simulink model "SMC_ISTSMC_ATSMC_IASMC_Leukemia_nonmono"  (R2024b)
settings: Solver=VariableStepAuto  StartTime=0.0  StopTime=20  RelTol=1e-3  EnableMultiTasking=on
undefined symbols (not defined in the file or in its folder): DiscIntNeverNeededParam
settings Model: Creator=engry  LastModifiedBy=munir
settings SolverCC: DateTimeAtSimulationTimeZero=[]  AlgebraicLoopSolver=TrustRegion
settings DataIOCC: ReturnWorkspaceOutputs=off
settings OptimizationCC: LifeSpan=inf
settings DebuggingCC: UnconnectedInputMsg=warning  UnconnectedOutputMsg=warning  UnconnectedLineMsg=warning  SFUnexpectedBacktrackingDiag=warning  SFNoUnconditionalDefaultTransitionDiag=warning  ArithmeticOperatorsInVariantConditions=warning
settings ModelReferenceCC: EnableRefExpFcnMdlSchedulingChecks=on
settings SFSimCC: SimUseLocalCustomCode=off  CustomCodeUndefinedFunction=UseInterfaceOnly
settings RTWCC: RTWUseLocalCustomCode=off  GPUComputeCapability=3.5
settings CodeAppCC: StateflowObjectComments=on
settings GRTTargetCC: TargetLangStandard=C89/C90 (ANSI)
settings ConfigComp: CovMetricSettings=dw  CovSaveCumulativeToWorkspaceVar=on  CovSaveSingleToWorkspaceVar=on  CovExternalEMLEnable=off

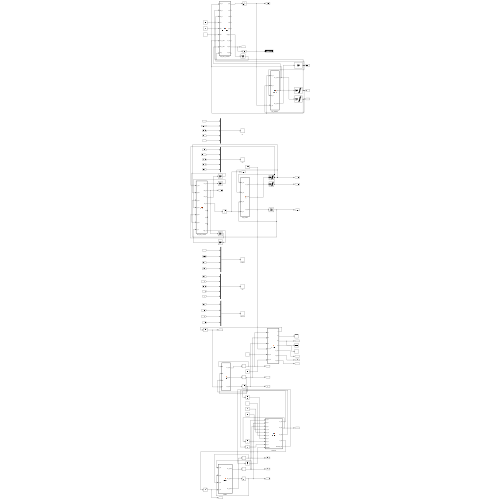
[thumbnail: Simulink's stored preview of the top-level diagram]
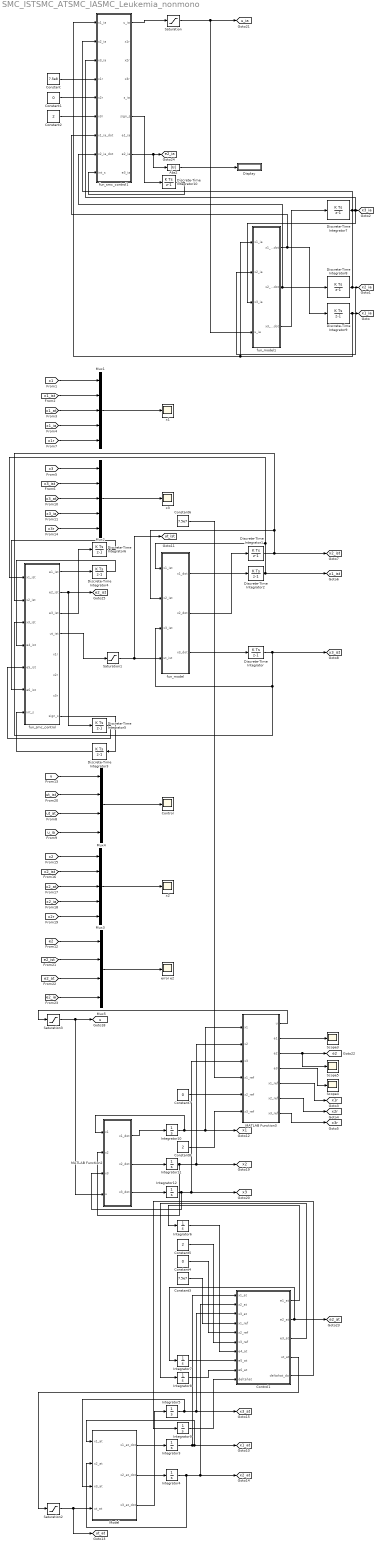
== system SMC_ISTSMC_ATSMC_IASMC_Leukemia_nonmono ==
  Abs2 : Abs  SaturateOnIntegerOverflow=off
  Constant : Constant  Value=7.5e8
  Constant1 : Constant  Value=0
  Constant2 : Constant  Value=2
  Constant3 : Constant  Value=7.5e7
  Constant4 : Constant  Value=0
  Constant5 : Constant  Value=2
  Constant6 : Constant  Value=7.5e7
  Constant7 : Constant  Value=0
  Constant8 : Constant  Value=2
  Control : Scope
  Control1 : MATLAB Function  TreatAsAtomicUnit=on  SystemSampleTime=0.01
  Discrete-Time Integrator : DiscreteIntegrator  SampleTime=-1  LowerSaturationLimit=0  ICPrevOutput=DiscIntNeverNeededParam  ICPrevScaledInput=DiscIntNeverNeededParam
  Discrete-Time Integrator1 : DiscreteIntegrator  InitialCondition=1e8  SampleTime=-1  LimitOutput=on  LowerSaturationLimit=0  ICPrevOutput=DiscIntNeverNeededParam  ICPrevScaledInput=DiscIntNeverNeededParam
  Discrete-Time Integrator10 : DiscreteIntegrator  SampleTime=-1  LowerSaturationLimit=0  ICPrevOutput=DiscIntNeverNeededParam  ICPrevScaledInput=DiscIntNeverNeededParam
  Discrete-Time Integrator2 : DiscreteIntegrator  InitialCondition=1.8e8  SampleTime=-1  LimitOutput=on  LowerSaturationLimit=7.5e7  ICPrevOutput=DiscIntNeverNeededParam  ICPrevScaledInput=DiscIntNeverNeededParam
  Discrete-Time Integrator{3..6} (4 alike) : DiscreteIntegrator  SampleTime=-1  ICPrevOutput=DiscIntNeverNeededParam  ICPrevScaledInput=DiscIntNeverNeededParam
  Discrete-Time Integrator7 : DiscreteIntegrator  SampleTime=-1  UpperSaturationLimit=2  LowerSaturationLimit=0  ICPrevOutput=DiscIntNeverNeededParam  ICPrevScaledInput=DiscIntNeverNeededParam
  Discrete-Time Integrator8 : DiscreteIntegrator  InitialCondition=1e8  SampleTime=-1  LimitOutput=on  LowerSaturationLimit=0  ICPrevOutput=DiscIntNeverNeededParam  ICPrevScaledInput=DiscIntNeverNeededParam
  Discrete-Time Integrator9 : DiscreteIntegrator  InitialCondition=1.8e8  SampleTime=-1  LimitOutput=on  LowerSaturationLimit=7.5e7  ICPrevOutput=DiscIntNeverNeededParam  ICPrevScaledInput=DiscIntNeverNeededParam
  Display : Display
  Integrator10 : Integrator  InitialCondition=1e8  LimitOutput=on  LowerSaturationLimit=7.5e7
  Integrator11 : Integrator  InitialCondition=1.8e8  LimitOutput=on  LowerSaturationLimit=0
  Integrator12 : Integrator  LimitOutput=on  UpperSaturationLimit=2  LowerSaturationLimit=0
  Integrator3 : Integrator  InitialCondition=1.8e8  LimitOutput=on  LowerSaturationLimit=7.5e7  ZeroCross=off
  Integrator4 : Integrator  InitialCondition=1e8  LimitOutput=on  LowerSaturationLimit=0
  Integrator5 : Integrator  ZeroCross=off
  Integrator{6..9} (4 alike) : Integrator
  MATLAB Function2 : MATLAB Function  TreatAsAtomicUnit=on
  MATLAB Function3 : MATLAB Function  TreatAsAtomicUnit=on
  Model : MATLAB Function  TreatAsAtomicUnit=on
  Mux1 : Mux  Inputs=5
  Mux2 : Mux  Inputs=5
  Mux3 : Mux  Inputs=5
  Mux4 : Mux
  Mux5 : Mux
  Saturation : Saturate  UpperLimit=1  LowerLimit=0
  Saturation1 : Saturate  UpperLimit=1  LowerLimit=0
  Saturation2 : Saturate  UpperLimit=1  LowerLimit=0  ZeroCross=off  RndMeth=Ceiling
  Saturation3 : Saturate  UpperLimit=1  LowerLimit=0  ZeroCross=off  RndMeth=Ceiling
  Scope3 : Scope
  Scope4 : Scope
  Scope5 : Scope
  error e2 : Scope
  fun_model : MATLAB Function  TreatAsAtomicUnit=on
  fun_model1 : MATLAB Function  TreatAsAtomicUnit=on
  fun_smc_control : MATLAB Function  TreatAsAtomicUnit=on
  fun_smc_control1 : MATLAB Function  TreatAsAtomicUnit=on
  x1 : Scope
  x2 : Scope
  x3 : Scope
  tag scope: e2=global, e2_at=global, e2_ia=global, e2_ist=global, u=global, u_ia=global, ut_at=global, ut_ist=global, x1=global, x1_at=global, x1_ia=global, x1_ist=global, x1r=global, x2=global, x2_at=global, x2_ia=global, x2_ist=global, x2r=global, x3=global, x3_at=global, x3_ia=global, x3_ist=global, x3r=global
  wires:
  Constant/1 -> fun_smc_control1/4("x1r ")
  Saturation2/1 -> [ut_at], Model/4(ut_at)
  fun_model/1(x1_dot) -> Discrete-Time Integrator2/1
  [x3_ia] -> Mux2/4
  Integrator7/1 -> Control1/8(e5_at)
  [x1] -> Mux1/1
  fun_model/3(x3_dot) -> Discrete-Time Integrator/1
  Constant1/1 -> fun_smc_control1/5("x2r ")
  Constant6/1 -> MATLAB Function3/4("x1_ref ")
  Constant2/1 -> fun_smc_control1/6("x3r ")
  Mux2/1 -> x3/1
  fun_smc_control/8(sign_s) -> Discrete-Time Integrator3/1
  [x3r] -> Mux2/5
  [x1_ist] -> Mux1/2
  [e2_at] -> Mux5/3
  [x1_at] -> Mux1/3
  [e2_ia] -> Mux5/4
  [x1_ia] -> Mux1/4
  Control1/5(deltahat_dot) -> Integrator9/1
  [u_ia] -> Mux4/4
  [x1r] -> Mux1/5
  [ut_ist] -> Mux4/2
  [x3] -> Mux2/1
  Integrator10/1 -> MATLAB Function3/1(x1), [x1], MATLAB Function2/1(x1)
  [x3_ist] -> Mux2/2
  [e2] -> Mux5/1
  [x3_at] -> Mux2/3
  fun_smc_control1/6(sign_s) -> Discrete-Time Integrator10/1
  fun_smc_control/1(e1_ist) -> Discrete-Time Integrator4/1
  [e2_ist] -> Mux5/2
  fun_smc_control/2(e2_ist) -> [e2_ist], Discrete-Time Integrator5/1
  fun_smc_control/3(e3_ist) -> Discrete-Time Integrator6/1
  fun_smc_control/4(ut_ist) -> Saturation1/1
  [u] -> Mux4/1
  Mux4/1 -> Control/1
  Discrete-Time Integrator4/1 -> fun_smc_control/4(e4_ist)
  [x2] -> Mux3/1
  [x2r] -> Mux3/5
  MATLAB Function3/2(e1) -> Scope3/1
  [ut_at] -> Mux4/3
  Saturation1/1 -> [ut_ist], fun_model/4(ut_ist)
  Discrete-Time Integrator6/1 -> fun_smc_control/6(e6_ist)
  [x2_ia] -> Mux3/4
  [x2_ist] -> Mux3/2
  [x2_at] -> Mux3/3
  Discrete-Time Integrator5/1 -> fun_smc_control/5(e5_ist)
  Saturation3/1 -> MATLAB Function2/4(u), [u]
  Mux5/1 -> error e2/1
  Discrete-Time Integrator3/1 -> fun_smc_control/7(int_s)
  Saturation/1 -> fun_model1/4(u_ia), [u_ia]
  fun_smc_control1/1(u_ia) -> Saturation/1
  Mux3/1 -> x2/1
  fun_smc_control1/8(e2_ia) -> [e2_ia], Abs2/1
  Discrete-Time Integrator10/1 -> fun_smc_control1/9(int_s)
  Mux1/1 -> x1/1
  MATLAB Function2/1(x1_dot) -> Integrator10/1
  MATLAB Function2/2(x2_dot) -> Integrator11/1
  Integrator9/1 -> Control1/10(deltahat)
  MATLAB Function2/3(x3_dot) -> Integrator12/1
  Model/1(x1_at_dot) -> Integrator3/1
  Model/2(x2_at_dot) -> Integrator4/1
  Constant7/1 -> MATLAB Function3/5("x2_ref ")
  Model/3(x3_at_dot) -> Integrator5/1
  Abs2/1 -> Display/1
  fun_model/2(x2_dot) -> Discrete-Time Integrator1/1
  Constant8/1 -> MATLAB Function3/6("x3_ref ")
  Integrator11/1 -> MATLAB Function3/2(x2), [x2], MATLAB Function2/2(x2)
  Integrator12/1 -> MATLAB Function3/3(x3), [x3], MATLAB Function2/3(x3)
  Integrator6/1 -> Control1/7(e4_at)
  Constant5/1 -> Control1/6(x3_ref)
  Constant4/1 -> Control1/5(x2_ref)
  Constant3/1 -> Control1/4(x1_ref)
  Integrator8/1 -> Control1/9(e6_at)
  MATLAB Function3/4(e3) -> Scope4/1
  Integrator5/1 -> [x3_at], Control1/3(x3_at), Model/3(x3_at)
  Integrator3/1 -> Model/1(x1_at), [x1_at], Control1/1(x1_at)
  Integrator4/1 -> [x2_at], Control1/2(x2_at), Model/2(x2_at)
  fun_model1/1(x1_ia_dot) -> fun_smc_control1/7(x1_ia_dot), Discrete-Time Integrator9/1
  fun_model1/2(x2_ia_dot) -> fun_smc_control1/8(x2_ia_dot), Discrete-Time Integrator8/1
  fun_model1/3(x3_ia_dot) -> Discrete-Time Integrator7/1
  Discrete-Time Integrator1/1 -> fun_smc_control/2(x2_ist), fun_model/2(x2_ist), [x2_ist]
  Discrete-Time Integrator2/1 -> fun_model/1(x1_ist), fun_smc_control/1(x1_ist), [x1_ist]
  Discrete-Time Integrator/1 -> fun_smc_control/3(x3_ist), fun_model/3(x3_ist), [x3_ist]
  MATLAB Function3/1(u) -> Saturation3/1
  MATLAB Function3/3(e2) -> [e2], Scope5/1
  MATLAB Function3/5(x1_ref) -> [x1r]
  MATLAB Function3/6(x2_ref) -> [x2r]
  MATLAB Function3/7(x3_ref) -> [x3r]
  Control1/1(e1_at) -> Integrator6/1
  Control1/2(e2_at) -> Integrator7/1, [e2_at]
  Control1/3(e3_at) -> Integrator8/1
  Control1/4(ut_at) -> Saturation2/1
  Discrete-Time Integrator7/1 -> fun_smc_control1/3(x3_ia), fun_model1/3(x3_ia), [x3_ia]
  Discrete-Time Integrator8/1 -> fun_smc_control1/2(x2_ia), [x2_ia], fun_model1/2(x2_ia)
  Discrete-Time Integrator9/1 -> fun_model1/1(x1_ia), fun_smc_control1/1(x1_ia), [x1_ia]

== matlab function SMC_ISTSMC_ATSMC_IASMC_Leukemia_nonmono/Model ==
  data: x1_at input; x1_at_dot output; x2_at input; x3_at input; x2_at_dot output; x3_at_dot output; ut_at input
function[x1_at_dot, x2_at_dot, x3_at_dot] = system(x1_at, x2_at, x3_at, ut_at)

r_l = 0.1;
r_n = 0.1;
lambda_l = 1.4;
lambda_n = 2.5;
La = 1e10;
Na = 1e10;
d = 0.4;
m1 = 0.04;
m2 = 0.04;
c = 1e-10;
b1=0.01;
b2=0.01;

%/------------System Model-----------------------%
x1_at_dot = (r_n * x1_at *log(Na))-(r_n*x1_at*real(log(complex(x1_at))))-((c*x1_at*x2_at)/(1+x2_at))-(m1*x1_at)-(lambda_n*x1_at*x3_at)+(b1*lambda_n*x1_at*x3_at^2);
x2_at_dot = (r_l*x2_at *log(La))-(r_l*x2_at*real(log(complex(x2_at))))-(m2 * x2_at)-(lambda_l*x2_at*x3_at)+(b2*lambda_l*x2_at*x3_at^2);
x3_at_dot = (-d * x3_at) + ut_at;

== matlab function SMC_ISTSMC_ATSMC_IASMC_Leukemia_nonmono/MATLAB Function2 ==
  data: x1 input; x1_dot output; x2 input; x3 input; x2_dot output; x3_dot output; u input
function[x1_dot, x2_dot, x3_dot] = syste(x1, x2, x3, u)

r_l = 0.1;
r_n = 0.1;
lambda_l = 2.5;
lambda_n = 1.4;
La = 1e10;
Na = 1e10;
d = 0.4;
m1 = 0.04;
m2 = 0.04;
c = 1e-1;
b1=0.01;
b2=0.01;

%System Model
x1_dot = r_n * x1 *log(Na) - r_n*x1*real(log(complex(x1))) - m1*x1 - (c*x1*x2)/(1+x2)-lambda_n*x1*(x3 - b1*x3^2);

x2_dot = r_l*x2 *log(La) - r_l*x2*real(log(complex(x2))) - m2*x2 - lambda_l*x2*(x3-b2*x3^2);

x3_dot = -d*x3 + u;

== matlab function SMC_ISTSMC_ATSMC_IASMC_Leukemia_nonmono/MATLAB Function3 ==
  data: u output; e1 output; e2 output; e3 output; x1 input; x2 input; x3 input; x1_ref input; x2_ref input; x3_ref input; x1_ref output; x2_ref output; x3_ref output
function [u,e1,e2,e3,x1_ref,x2_ref,x3_ref]=control(x1,x2,x3,x1_ref,x2_ref,x3_ref)

r_l = 0.1;
r_n = 0.1;
lambda_l = 2.5;
lambda_n = 1.4;
La = 1e10;
Na = 1e10;
d = 0.4;
m1 = 0.04; %gamma_n
m2 = 0.04; %%gamma_l
c = 1e-1;
b1=0.01;
b2=0.01;

x1_dot = r_n * x1 *log(Na) - r_n*x1*real(log(complex(x1))) - m1*x1 - (c*x1*x2)/(1+x2)-lambda_n*x1*(x3 - b1*x3^2);

x2_dot = r_l*x2 *log(La) - r_l*x2*real(log(complex(x2))) - m2*x2 - lambda_l*x2*(x3-b2*x3^2);



a1=1e-15;
a2=1e-15;
a3=0.1;
alpha=0.95;
phi=0.75;
k=1;

e1=x1-x1_ref;
e2=x2-x2_ref;
e3=x3-x3_ref;

s=a1*e1+a2*e2+a3*e3;

u=(-k*((abs(s))^alpha)*(sign(s/phi))/a3) - (a1*x1_dot/a3) - (a2*x2_dot/a3) + (d*x3);

== matlab function SMC_ISTSMC_ATSMC_IASMC_Leukemia_nonmono/fun_smc_control1 ==
  data: u_ia output; x1r output; x2r output; x3r output; s_ia output; x1_ia input; x2_ia input; x3_ia input; x1r input; x2r input; x3r input; x1_ia_dot input; x2_ia_dot input; sign_s output; int_s input; e1_ia output; e2_ia output; e3_ia output
function [u_ia, x1r,x2r,x3r,s_ia,sign_s,e1_ia,e2_ia,e3_ia] = cont_iasmc(x1_ia, x2_ia, x3_ia, x1r,x2r,x3r,x1_ia_dot, x2_ia_dot, int_s)
% Impulsive Adaptive Sliding Mode Control

% Parameters
gh = 0.4;

alpha = 0.5;

v1=1e-16; 
v2=1e-16; 
v3=0.95;

c1=9e-1;
c2=9e-1;


% errors
e1_ia = x1_ia-x1r;                               
e2_ia = x2_ia-x2r;    
e3_ia = x3_ia-x3r; 

% sliding surface
s_ia = v1*e1_ia+v2*e2_ia+v3*e3_ia;

sign_s = sign(s_ia);

dot_x1_ref = 0;
dot_x2_ref = 0;
dot_x3_ref = 0;

beta = 1e-2;
rho0 = 1e-2;
s_th = 1e-1;
t = 1;
tk_array = [t; t+1];

Simp = rho0*(1+beta*abs(sign(s_ia)));
Impulsive = Simp*sign(s_ia);

if abs(s_ia) > s_th && any(abs(t - tk_array) < 1e-4) % impulse at t ≈ tk
delta_uk = Impulsive;
else
delta_uk = 0;
end

% control inputs
u_eq = gh*x3_ia + dot_x3_ref -(v1/v3)*(x1_ia_dot-dot_x1_ref)-(v2/v3)*(x2_ia_dot-dot_x2_ref);

u_sw = -c1*(abs(s_ia))^alpha*(sign(s_ia))-c2*(int_s);

% final control input
u_ia = u_eq + u_sw + delta_uk;

== matlab function SMC_ISTSMC_ATSMC_IASMC_Leukemia_nonmono/fun_model1 ==
  data: x1_ia_dot output; x2_ia_dot output; x1_ia input; x2_ia input; x3_ia input; u_ia input; x3_ia_dot output
function [x1_ia_dot, x2_ia_dot, x3_ia_dot] = model(x1_ia,x2_ia,x3_ia,u_ia)
% Initial values x1_0 = 1.8e8;x2_0 = 1e8;x3_0 = 0;u_max = 1; x1_min = 7.5e+7;

% Parameters
rn = 0.1; 
rl = 0.1;
gn = 0.04; 
gl = 0.04;
gh = 0.4;
La = 1e+10;
Na = 1e+10;

a1 = 0.01;
a2 = 0.01;

c = 1e-1;

lambda_l = 1.4;
lambda_n = 2.5;

%% Leukemia mathematical model with non-monotonic therapy 
% Note: (x1*x3)/(a1*(x3)^2+(b1)*x3+1) ~ x1*x3 - a1*x1*x3^2

x1_ia_dot = rn*x1_ia*log(Na) - rn*x1_ia*real(log(complex(x1_ia))) - gn*x1_ia - (c*x1_ia*x2_ia)/(1+x2_ia) - lambda_n*x1_ia*(x3_ia - a1*x3_ia^2);
x2_ia_dot = rl*x2_ia*log(La) - rl*x2_ia*real(log(complex(x2_ia))) - gl*x2_ia - lambda_l*x2_ia*(x3_ia - a2*x3_ia^2);
x3_ia_dot = -gh*x3_ia + u_ia;

== matlab function SMC_ISTSMC_ATSMC_IASMC_Leukemia_nonmono/fun_model ==
  data: x1_dot output; x2_dot output; x1_ist input; x2_ist input; x3_ist input; ut_ist input; x3_dot output
function [x1_dot, x2_dot, x3_dot] = model(x1_ist,x2_ist,x3_ist,ut_ist)
% Initial values x1_0 = 1.8e8;x2_0 = 1e8;x3_0 = 0;u_max = 1; x1_min = 7.5e+7;

% Parameters
rn = 0.1; 
rl = 0.1;
gn = 0.04; 
gl = 0.04;
gh = 0.4;
La = 1e+10;
Na = 1e+10;

b1 = 0.01;
b2 = 0.01;

c = 1e-2;

lambda_n = 2.5;
lambda_l = 1.4;

%% Leukemia mathematical model with non-monotonic therapy 
x1_dot = (rn*x1_ist*log(Na))-(rn*x1_ist*real(log(complex(x1_ist))))-((c*x1_ist*x2_ist)/(1+x2_ist))-(gn*x1_ist)-(lambda_n*x1_ist*x3_ist)+(b1*lambda_n*x1_ist*x3_ist^2);
x2_dot = (rl*x2_ist*log(La))-(rl*x2_ist*real(log(complex(x2_ist))))-(gl*x2_ist)-(lambda_l*x2_ist*x3_ist)+(b2*lambda_l*x2_ist*x3_ist^2);

x3_dot = -gh*x3_ist + ut_ist;

== matlab function SMC_ISTSMC_ATSMC_IASMC_Leukemia_nonmono/fun_smc_control ==
  data: e1_ist output; e2_ist output; e3_ist output; x1_ist input; ut_ist output; x2_ist input; x3_ist input; e4_ist input; e5_ist input; e6_ist input; x1r output; x2r output; x3r output; int_s input; sign_s output
function [e1_ist,e2_ist,e3_ist,ut_ist,x1r,x2r,x3r,sign_s] = cont_istsmc(x1_ist, x2_ist, x3_ist, e4_ist,e5_ist,e6_ist, int_s)
%Sliding Mode Control

% Parameters
rn = 0.1; 
rl = 0.1;
gn = 0.04; 
gl = 0.04;
gh = 0.4;
La = 1e10;
Na = 1e10;

a1 = 0.01;
b1 = 0.0;
a2 = 0.01;
b2 = 0.0;

c = 1e-2;

alpha = 1e-0;

lambda_l = 1.4;
lambda_n = 2.5;

v1=1e-15; 
v2=1e-15; 
v3=0.2;

k1=1e-15; 
k2=1e-15; 
k3=0.1;

c1=1e-1;
c2=0.5227;

% reference values
x1r = 7.5e7;
x2r = 0;
x3r = 2;

lambda_n = 2.5;
lambda_l = 1.4;


% errors
e1_ist = (x1_ist-x1r);                               
e2_ist = (x2_ist-x2r);    
e3_ist = (x3_ist-x3r); 

% sliding surface
s = (v1*e1_ist+v2*e2_ist+v3*e3_ist)+(k1*e4_ist+k2*e5_ist+k3*e6_ist);

sign_s = sign(s);

x1_dot = (rn * x1_ist *log(Na))-(rn*x1_ist*real(log(complex(x1_ist))))-((c*x1_ist*x2_ist)/(1+x2_ist))-(gn*x1_ist)-(lambda_n*x1_ist*x3_ist)+(b1*lambda_n*x1_ist*x3_ist^2);
x2_dot = (rl*x2_ist *log(La))-(rl*x2_ist*real(log(complex(x2_ist))))-(gl*x2_ist)-(lambda_l*x2_ist*x3_ist)+(b2*lambda_l*x2_ist*x3_ist^2);

%% control under non-monotonic
ut_ist = gh*x3_ist - (v1/v3)*(x1_dot - 0) - (v2/v3)*(x2_dot - 0) - (v1*e1_ist+v2*e2_ist+v3*e3_ist)/v3 - c1*(abs(s))^(alpha)*sign(s) - c2*int_s;

== matlab function SMC_ISTSMC_ATSMC_IASMC_Leukemia_nonmono/Control1 ==
  data: e1_at output; e2_at output; e3_at output; ut_at output; x1_at input; x2_at input; x3_at input; x1_ref input; x2_ref input; x3_ref input; e4_at input; e5_at input; e6_at input; deltahat input; deltahat_dot output
function [e1_at, e2_at, e3_at, ut_at, deltahat_dot] = control(x1_at, x2_at, x3_at, x1_ref, x2_ref, x3_ref, e4_at, e5_at, e6_at, deltahat)


% === Model Parameters ===
r_l = 0.1;
r_n = 0.1;
lambda_l = 1.4;
lambda_n = 2.5;
La = 1e10;
Na = 1e10;
d = 0.4;
m1 = 0.04;
m2 = 0.04;
c = 1e-10;
b1=0.01;
b2=0.01;

% === TSMC Control Gains ===
a1 = 1e-15;   % Gain for e1 (normal cell error) 
a2 = 1e-30;   % Gain for e2 (leukemic cell error) 
a3 = 100;    % Gain for e3 (chemo error) 
a4 = 1e-15;   % Gain for int_e1 (normal cell integral)
a5 = 1e-10;   % Gain for int_e2 (leukemic cell integral) 
a6 = 4000;    % Gain for int_e3 (chemo agent integral) 
alpha = 0.92; 
phi = 0.095; 
k = 25;      % Reduced for smoother u(t) 

% === Reference Errors ===
e1_at = x1_at - x1_ref;
e2_at = x2_at - x2_ref;
e3_at = x3_at - x3_ref;

% === Terminal Exponents ===
%p1=3;
%p2=3;
%p3=5;
%q1=3;
%q2=3;
%q3=5;

gg= 1.099;
hh= 1.09;
ii= 1.03;

% === State Derivatives ===
x1_at_dot = (r_n * x1_at *log(Na))-(r_n*x1_at*real(log(complex(x1_at))))-((c*x1_at*x2_at)/(1+x2_at))-(m1*x1_at)-(lambda_n*x1_at*x3_at)+(b1*lambda_n*x1_at*x3_at^2);
x2_at_dot = (r_l*x2_at *log(La))-(r_l*x2_at*real(log(complex(x2_at))))-(m2 * x2_at)-(lambda_l*x2_at*x3_at)+(b2*lambda_l*x2_at*x3_at^2);

% === Adaptive Terminal Sliding Surface ===
%s =a1*e1 + a2*e2 + a3*e3 + a4*e4^gg + a5*e5^hh + a6*e6^ii;
s = a1*e1_at + a2*e2_at + a3*e3_at + a4*real((complex(e4_at))^gg) + a5*real((complex(e5_at))^hh) + a6*real((complex(e6_at))^ii);


 eta= 0.0001 ;

%deltahat_dot = eta * a2 * x2 * s * log(La / x2);
deltahat_dot = eta * a2 * x2_at * s * log(La / real((complex(x2_at))));

% === Adaptive Terminal SMC Control Input ===


ut_at = (1/a3) * ( -k * abs(s)^alpha * sign(s / phi) - a1*x1_at_dot - a2*(deltahat*x2_at*log(La) - r_l*x2_at*real(log(complex(x2_at))) - ...
    m2*x2_at - lambda_l*x2_at*x3_at + b2*lambda_l*x2_at*x3_at^2) ... 
    - gg*a4*e1_at*real((complex(e4_at))^(gg - 1)) - hh*a5*e2_at*real((complex(e5_at))^(hh - 1)) ...
    - ii*a6*e3_at*real((complex(e6_at))^(ii - 1)) ) + d*x3_at;
